simulink model "InkrementalisDoc"  (R2013b)
settings: Solver=ode45  StartTime=0.0  StopTime=15  RelTol=1e-3
values from neighbouring files (symbols this model uses):
  duty = (dk-vd)/dk*100    (= 42.7042204869)    [incrementalis.m]
  periodus = dk    (= 1.0471975512)    [incrementalis.m]
settings Model: Creator=laca  LastModifiedBy=laca
settings DataIOCC: SignalLoggingSaveFormat=ModelDataLogs
settings DebuggingCC: UnderspecifiedInitializationDetection=Simplified  MultiTaskDSMMsg=warning  MultiTaskCondExecSysMsg=none
settings RTWCC: IncludeERTFirstTime=on
settings GRTTargetCC: CodeReplacementLibrary=None  CPPClassGenCompliant=on

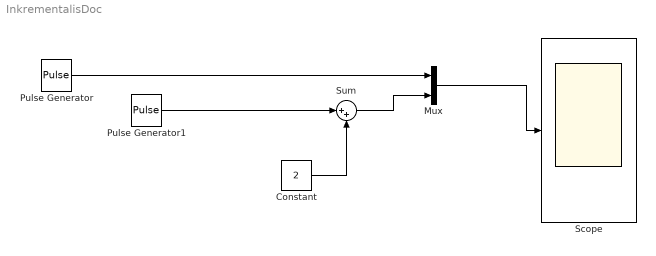
== system InkrementalisDoc ==
  Constant : Constant  Value=2
  Mux : Mux  Inputs=2
  Pulse Generator : DiscretePulseGenerator  PulseType=Time based  Period=periodus  PulseWidth=duty
  Pulse Generator1 : DiscretePulseGenerator  PulseType=Time based  Period=periodus  PulseWidth=duty  PhaseDelay=0.3
  Scope : Scope
  Sum : Sum  Inputs=|++
  wires:
  Mux/1 -> Scope/1
  Pulse Generator/1 -> Mux/1
  Pulse Generator1/1 -> Sum/1
  Constant/1 -> Sum/2
  Sum/1 -> Mux/2
